simulink model "ABCD_lat"  (R2025b)
settings: Solver=VariableStepAuto  StartTime=0.0  StopTime=10.0  RelTol=1e-3
values from neighbouring files (symbols this model uses):
  A_lat = A_full([3 4 6 7], [3 4 6 7])    [drl_simplified_dynamics.m]
  B_lat = B_full([3 4 6 7], [1 3])    [drl_simplified_dynamics.m]
undefined symbols (not defined in the file or in its folder): C_lat, D_lat
settings Model: Creator=19894  LastModifiedBy=19894

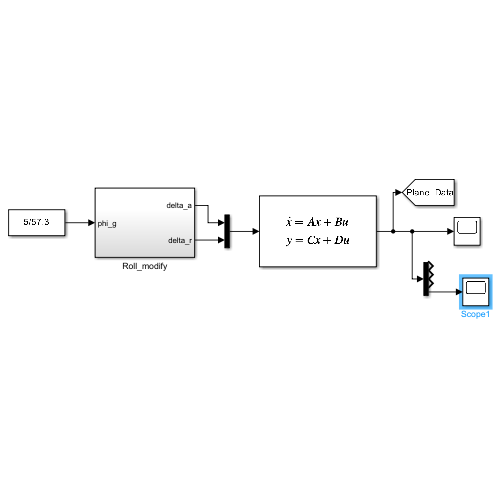
[thumbnail: Simulink's stored preview of the top-level diagram]
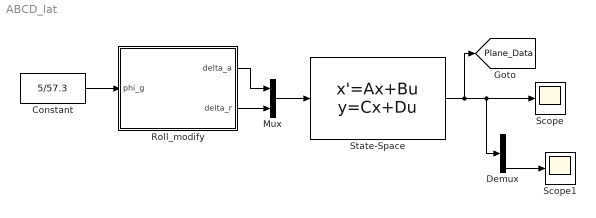
== system ABCD_lat ==
  Constant : Constant  Value=5/57.3
  Demux : Demux
  Mux : Mux  Inputs=2
  Roll_modify : Subsystem
  Scope : Scope
      settings: ActiveDisplayYMinimum=-0.1237601749645708  ActiveDisplayYMaximum=1.1138208486177197
  Scope1 : Scope
      settings: ActiveDisplayYMinimum=-0.1237601749645708  ActiveDisplayYMaximum=1.1138208486177197
  State-Space : StateSpace  A=A_lat  B=B_lat  C=C_lat  D=D_lat  InitialCondition=0
  tag scope: Plane_Data=global
  wires:
  Roll_modify/1(delta_a) -> Mux/1
  Roll_modify/2(delta_r) -> Mux/2
  Mux/1 -> State-Space/1
  Constant/1 -> Roll_modify/1(phi_g)
  State-Space/1 -> [Plane_Data], Demux/1, Scope/1
  Demux/4 -> Scope1/1

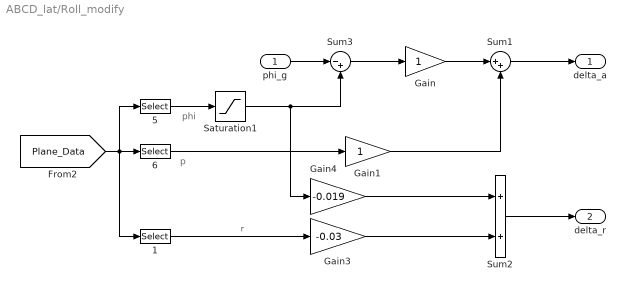
== system ABCD_lat/Roll_modify ==
  note: p
  note: phi
  phi_g : Inport
  1 : Selector  InputPortWidth=4  IndexOptions=Index vector (dialog)  Indices=3  OutputSizes=[(-2)]
  5 : Selector  InputPortWidth=4  IndexOptions=Index vector (dialog)  Indices=4  OutputSizes=[(-2)]
  6 : Selector  InputPortWidth=4  IndexOptions=Index vector (dialog)  Indices=2  OutputSizes=[(-2)]
  Gain : Gain
  Gain1 : Gain
  Gain3 : Gain  Gain=-0.03
  Gain4 : Gain  Gain=-0.019
  Saturation1 : Saturate  UpperLimit=30*pi/180  LowerLimit=-30*pi/180
  Sum1 : Sum  Inputs=|++
  Sum2 : Sum
  Sum3 : Sum  Inputs=|-+
  delta_a : Outport
  delta_r : Outport  Port=2
  wires:
  Sum1/1 -> delta_a/1
  Gain3/1 -> Sum2/2
  Gain4/1 -> Sum2/1
  Sum2/1 -> delta_r/1
  Sum3/1 -> Gain/1
  Gain/1 -> Sum1/1
  Saturation1/1 -> Gain4/1, Sum3/2
  [Plane_Data] -> 1/1, 6/1, 5/1
  1/1 -> Gain3/1  "r"
  6/1 -> Gain1/1
  phi_g/1 -> Sum3/1
  5/1 -> Saturation1/1
  Gain1/1 -> Sum1/2
